simulink library "sunSeek_lib"  (R2018b)
settings: Solver=VariableStepAuto  StartTime=0.0  StopTime=10.0  RelTol=1e-3
undefined symbols (not defined in the file or in its folder): fswParams
libraries: vrlib x1
settings Model: Creator=Taylor  LastModifiedBy=Taylor

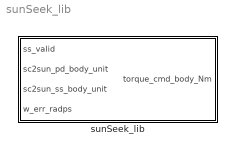
== system sunSeek_lib ==
  sunSeek_lib : Subsystem  TreatAsAtomicUnit=on
      settings: RTWSystemCode=Nonreusable function  RTWFcnNameOpts=Use subsystem name  RTWFileNameOpts=Use subsystem name

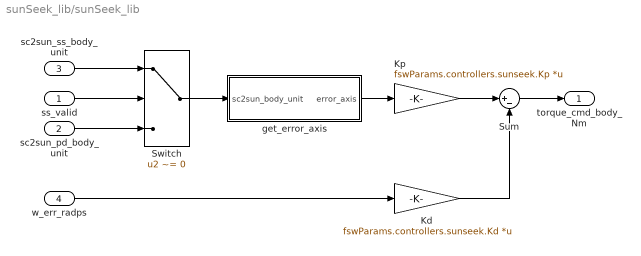
== system sunSeek_lib/sunSeek_lib ==
  ss_valid : Inport
  sc2sun_pd_body_unit : Inport  Port=2
  sc2sun_ss_body_unit : Inport  Port=3
  w_err_radps : Inport  Port=4
  Kd : Gain  Gain=fswParams.controllers.sunseek.Kd  Multiplication=Matrix(K*u) (u vector)
  Kp : Gain  Gain=fswParams.controllers.sunseek.Kp  Multiplication=Matrix(K*u) (u vector)
  Sum : Sum  Inputs=|+-
  Switch : Switch  Criteria=u2 ~= 0
  get_error_axis : Subsystem
  torque_cmd_body_Nm : Outport
  wires:
  ss_valid/1 -> Switch/2
  sc2sun_ss_body_unit/1 -> Switch/1
  sc2sun_pd_body_unit/1 -> Switch/3
  w_err_radps/1 -> Kd/1
  Kd/1 -> Sum/2
  Kp/1 -> Sum/1
  Sum/1 -> torque_cmd_body_Nm/1
  Switch/1 -> get_error_axis/1(sc2sun_body_unit)
  get_error_axis/1(error_axis) -> Kp/1

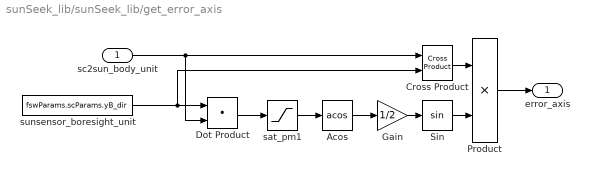
== system sunSeek_lib/sunSeek_lib/get_error_axis ==
  sc2sun_body_unit : Inport
  Acos : Trigonometry  Operator=acos
  Cross Product : vrlib/Utilities/Cross Product
      settings: SourceProductBaseCode=VR
  Dot Product : DotProduct  InputSameDT=on  OutDataTypeStr=Inherit: Inherit via internal rule
  Gain : Gain  Gain=1/2
  Product : Product
  Sin : Trigonometry
  sat_pm1 : Saturate  UpperLimit=1  LowerLimit=-1
  sunsensor_boresight_unit : Constant  Value=fswParams.scParams.yB_dir
  error_axis : Outport
  wires:
  Product/1 -> error_axis/1
  Cross Product/1 -> Product/1
  sat_pm1/1 -> Acos/1
  sc2sun_body_unit/1 -> Dot Product/2, Cross Product/1
  sunsensor_boresight_unit/1 -> Dot Product/1, Cross Product/2
  Acos/1 -> Gain/1
  Gain/1 -> Sin/1
  Sin/1 -> Product/2
  Dot Product/1 -> sat_pm1/1
